simulink model "sampleModel7126_pp_1_1"  (R2018a)
settings: Solver=VariableStepAuto  StartTime=0.0  StopTime=10.0  RelTol=1e-3
undefined symbols (not defined in the file): DiscIntNeverNeededParam
libraries: simulink x367
(part 2 of 12)

== system sampleModel7126_pp_1_1/cfblk15 ==
  emi_1747 : Inport
  Action Port : ActionPort  ActionType=then
  cfblk15 : simulink/Continuous/PID Controller  Controller=PID  TimeDomain=Discrete-time  SampleTime=1  IntegratorMethod=Forward Euler  FilterMethod=Forward Euler  Form=Parallel  UseFilter=on  ControllerParametersSource=internal  P=1  I=1  D=0  N=100  InitialConditionSource=internal  InitialConditionForIntegrator=0  InitialConditionForFilter=0  ExternalReset=none  LimitOutput=off  UpperSaturationLimit=inf  LowerSaturationLimit=-inf  LinearizeAsGain=off  AntiWindupMode=none  Kb=1  TrackingMode=off  Kt=1  PParamMin=[]  PParamMax=[]  IParamMin=[]  IParamMax=[]  DParamMin=[]  DParamMax=[]  NParamMin=[]  NParamMax=[]  KbParamMin=[]  KbParamMax=[]  KtParamMin=[]  KtParamMax=[]  POutMin=[]  POutMax=[]  IOutMin=[]  IOutMax=[]  DOutMin=[]  DOutMax=[]  NOutMin=[]  NOutMax=[]  KbOutMin=[]  KbOutMax=[]  KtOutMin=[]  KtOutMax=[]  IntegratorOutMin=[]  IntegratorOutMax=[]  FilterOutMin=[]  FilterOutMax=[]  SumOutMin=[]  SumOutMax=[]  SumI1OutMin=[]  SumI1OutMax=[]  SumI2OutMin=[]  SumI2OutMax=[]  SumI3OutMin=[]  SumI3OutMax=[]  SumDOutMin=[]  SumDOutMax=[]  SaturationOutMin=[]  SaturationOutMax=[]  IntegratorContinuousStateAttributes=''  IntegratorStateMustResolveToSignalObject=off  IntegratorRTWStateStorageClass=Auto  FilterContinuousStateAttributes=''  FilterStateMustResolveToSignalObject=off  FilterRTWStateStorageClass=Auto  DifferentiatorICPrevScaledInput=0  DifferentiatorOutMin=[]  DifferentiatorOutMax=[]  FilterDiffOutCoefMin=[]  FilterDiffOutCoefMax=[]  SumDenOutMin=[]  SumDenOutMax=[]  SumNumOutMin=[]  SumNumOutMax=[]  ReciprocalOutMin=[]  ReciprocalOutMax=[]  DivideOutMin=[]  DivideOutMax=[]  TunerSelectOption=Transfer Function Based (PID Tuner App)
  emi_1748 : Outport
  wires:
  emi_1747/1 -> cfblk15/1
  cfblk15/1 -> emi_1748/1

== system sampleModel7126_pp_1_1/cfblk20 ==
  emi_1949 : Inport
  emi_1950 : Inport  Port=2
  Action Port : ActionPort  ActionType=then
  cfblk20 : Delay  DelayLengthSource=Input port  SampleTime=1
      settings: InputPortMap=u0,p1
  emi_1951 : Outport
  wires:
  emi_1949/1 -> cfblk20/1
  emi_1950/1 -> cfblk20/2
  cfblk20/1 -> emi_1951/1

== system sampleModel7126_pp_1_1/cfblk21 ==
  emi_194 : Inport
  emi_195 : Inport  Port=2
  Action Port : ActionPort  ActionType=then
  cfblk21 : simulink/Continuous/PID Controller (2DOF)  Controller=PID  TimeDomain=Discrete-time  SampleTime=1  IntegratorMethod=Forward Euler  FilterMethod=Forward Euler  Form=Parallel  UseFilter=on  ControllerParametersSource=internal  P=1  I=1  D=0  N=100  b=1  c=1  InitialConditionSource=internal  InitialConditionForIntegrator=0  InitialConditionForFilter=0  ExternalReset=none  LimitOutput=off  UpperSaturationLimit=inf  LowerSaturationLimit=-inf  LinearizeAsGain=off  AntiWindupMode=none  Kb=1  TrackingMode=off  Kt=1  PParamMin=[]  PParamMax=[]  IParamMin=[]  IParamMax=[]  DParamMin=[]  DParamMax=[]  NParamMin=[]  NParamMax=[]  bParamMin=[]  bParamMax=[]  cParamMin=[]  cParamMax=[]  KbParamMin=[]  KbParamMax=[]  KtParamMin=[]  KtParamMax=[]  POutMin=[]  POutMax=[]  IOutMin=[]  IOutMax=[]  DOutMin=[]  DOutMax=[]  NOutMin=[]  NOutMax=[]  bOutMin=[]  bOutMax=[]  cOutMin=[]  cOutMax=[]  KbOutMin=[]  KbOutMax=[]  KtOutMin=[]  KtOutMax=[]  IntegratorOutMin=[]  IntegratorOutMax=[]  FilterOutMin=[]  FilterOutMax=[]  SumOutMin=[]  SumOutMax=[]  Sum1OutMin=[]  Sum1OutMax=[]  Sum2OutMin=[]  Sum2OutMax=[]  Sum3OutMin=[]  Sum3OutMax=[]  SumI1OutMin=[]  SumI1OutMax=[]  SumI2OutMin=[]  SumI2OutMax=[]  SumI3OutMin=[]  SumI3OutMax=[]  SumDOutMin=[]  SumDOutMax=[]  SaturationOutMin=[]  SaturationOutMax=[]  IntegratorContinuousStateAttributes=''  IntegratorStateMustResolveToSignalObject=off  IntegratorRTWStateStorageClass=Auto  FilterContinuousStateAttributes=''  FilterStateMustResolveToSignalObject=off  FilterRTWStateStorageClass=Auto  DifferentiatorICPrevScaledInput=0  DifferentiatorOutMin=[]  DifferentiatorOutMax=[]  FilterDiffOutCoefMin=[]  FilterDiffOutCoefMax=[]  SumDenOutMin=[]  SumDenOutMax=[]  SumNumOutMin=[]  SumNumOutMax=[]  ReciprocalOutMin=[]  ReciprocalOutMax=[]  DivideOutMin=[]  DivideOutMax=[]  TunerSelectOption=Transfer Function Based (PID Tuner App)
  emi_196 : Outport
  wires:
  emi_194/1 -> cfblk21/1
  emi_195/1 -> cfblk21/2
  cfblk21/1 -> emi_196/1

== system sampleModel7126_pp_1_1/cfblk245 ==
  cfblk1 : Inport
  cfblk11 : Inport  Port=2
  cfblk12 : Inport  Port=3
  cfblk13 : Inport  Port=4
  cfblk14 : Inport  Port=5
  cfblk15 : Inport  Port=6
  Action Port : ActionPort  ActionType=then
  cfblk10 : If  SampleTime=1
  cfblk18 : Subsystem  TreatAsAtomicUnit=on
  cfblk19 : Subsystem  TreatAsAtomicUnit=on
  cfblk20 : Delay
  cfblk21 : DataTypeConversion  OutDataTypeStr=double
  cfblk3 : DiscreteIntegrator  SampleTime=-1  OutDataTypeStr=double  ICPrevOutput=DiscIntNeverNeededParam  ICPrevScaledInput=DiscIntNeverNeededParam
  cfblk4 : UnitDelay  SampleTime=-1
  cfblk5 : DiscreteZeroPole  Poles=[0 0.5]  Gain=1  SampleTime=-1
  cfblk6 : DiscreteFilter
  cfblk7 : simulink/Discrete/Transfer Fcn Real Zero  ZeroZ=0.75  ICPrevInput=0.0  DoSatur=off
      settings: SourceProductName=Simulink  SourceProductBaseCode=SL
  cfblk8 : Subsystem  TreatAsAtomicUnit=on
  cfblk9 : Delay
  cyemi_{68..70,79,90,92..98} (12 alike) : DataTypeConversion  OutDataTypeStr=double
  cyemi_91 : DataTypeConversion  OutDataTypeStr=fixdt('ufix32_En8')
  emi_671 : Subsystem  TreatAsAtomicUnit=on
  emi_673 : If  IfExpression=Inf <= u1  SampleTime=[1 0]
  emi_674 : DataTypeConversion  OutDataTypeStr=double
  cfblk2 : Outport
  cfblk16 : Outport  Port=2
  cfblk17 : Outport  Port=3
  wires:
  cfblk4/1 -> cfblk16/1, emi_674/1
  cfblk14/1 -> cfblk2/1
  cfblk18/3(cfblk11) -> cfblk17/1
  cfblk10/1 -> cfblk18/Action
  cfblk10/2 -> cfblk19/Action
  cyemi_68/1 -> cfblk10/1
  cfblk11/1 -> cyemi_68/1
  cyemi_69/1 -> cfblk18/1(cfblk1)
  cfblk15/1 -> cyemi_69/1
  cyemi_70/1 -> cfblk18/2(cfblk9)
  cfblk19/3(cfblk12) -> cyemi_70/1
  cyemi_79/1 -> cfblk19/1(cfblk1)
  cfblk3/1 -> cyemi_79/1
  cyemi_90/1 -> cfblk20/1
  cfblk18/2(cfblk10) -> cyemi_90/1
  cyemi_91/1 -> cfblk21/1
  cfblk1/1 -> cyemi_91/1
  cyemi_92/1 -> cfblk3/1
  cfblk20/1 -> cyemi_92/1
  cyemi_93/1 -> cfblk4/1
  cfblk7/1 -> cyemi_93/1
  cyemi_94/1 -> cfblk5/1
  cfblk21/1 -> cyemi_94/1
  cyemi_95/1 -> cfblk6/1
  cfblk19/1(cfblk2) -> cyemi_95/1
  cyemi_96/1 -> cfblk7/1
  cfblk18/1(cfblk2) -> cyemi_96/1
  cfblk19/2(cfblk11) -> cyemi_97/1
  cyemi_98/1 -> cfblk9/1
  cyemi_97/1 -> cfblk8/1(emi_669)
  cfblk8/1(emi_670) -> cyemi_98/1
  emi_673/1 -> cfblk8/Action
  emi_673/2 -> emi_671/Action
  emi_674/1 -> emi_673/1

== system sampleModel7126_pp_1_1/cfblk246 ==
  cfblk1 : Inport
  cfblk8 : Inport  Port=2
  Action Port : ActionPort  ActionType=else
  cfblk10 : Subsystem  TreatAsAtomicUnit=on
  cfblk11 : Delay
  cfblk3 : DiscreteFilter
  cfblk4 : Subsystem  TreatAsAtomicUnit=on
  cfblk5 : Subsystem  TreatAsAtomicUnit=on
  cfblk6 : simulink/Discrete/Transfer Fcn Lead or Lag  PoleZ=0.95  ZeroZ=0.75  ICPrevOutput=0.0  ICPrevInput=0.0  DoSatur=off
      settings: SourceProductName=Simulink  SourceProductBaseCode=SL
  cfblk7 : If  SampleTime=1
  cfblk9 : Subsystem  TreatAsAtomicUnit=on
  cyemi_{101..102,118..124} (9 alike) : DataTypeConversion  OutDataTypeStr=double
  emi_1864 : Subsystem  TreatAsAtomicUnit=on
  emi_1866 : If  IfExpression=0 <= u1  SampleTime=[1 0]
  emi_1867 : DataTypeConversion  OutDataTypeStr=double
  emi_515 : Subsystem  TreatAsAtomicUnit=on
  emi_517 : If  IfExpression=0 <= u1  SampleTime=[1 0]
  emi_518 : DataTypeConversion  OutDataTypeStr=double
  cfblk2 : Outport
  wires:
  cfblk6/1 -> cfblk2/1
  cfblk7/1 -> cfblk9/Action
  cfblk7/2 -> cfblk10/Action
  cyemi_101/1 -> cfblk10/1(cfblk1)
  cfblk11/1 -> cyemi_101/1
  cyemi_102/1 -> cfblk10/2(cfblk13)
  cfblk8/1 -> cyemi_102/1
  cyemi_118/1 -> cfblk11/1
  cyemi_119/1 -> cfblk3/1
  cfblk1/1 -> cyemi_119/1
  cfblk10/1(cfblk2) -> cyemi_120/1
  cfblk3/1 -> cyemi_121/1, emi_518/1
  cyemi_122/1 -> cfblk6/1
  cfblk10/3(cfblk15) -> cyemi_122/1
  cyemi_123/1 -> cfblk7/1
  cyemi_124/1 -> cfblk9/1(cfblk1)
  cfblk10/2(cfblk14) -> cyemi_124/1
  cyemi_120/1 -> cfblk4/1(emi_513)
  cfblk4/1(emi_514) -> cyemi_118/1, emi_1867/1
  emi_517/1 -> cfblk4/Action
  emi_517/2 -> emi_515/Action
  emi_518/1 -> emi_517/1
  cyemi_121/1 -> cfblk5/1(emi_1862)
  cfblk5/1(emi_1863) -> cyemi_123/1
  emi_1866/1 -> cfblk5/Action
  emi_1866/2 -> emi_1864/Action
  emi_1867/1 -> emi_1866/1

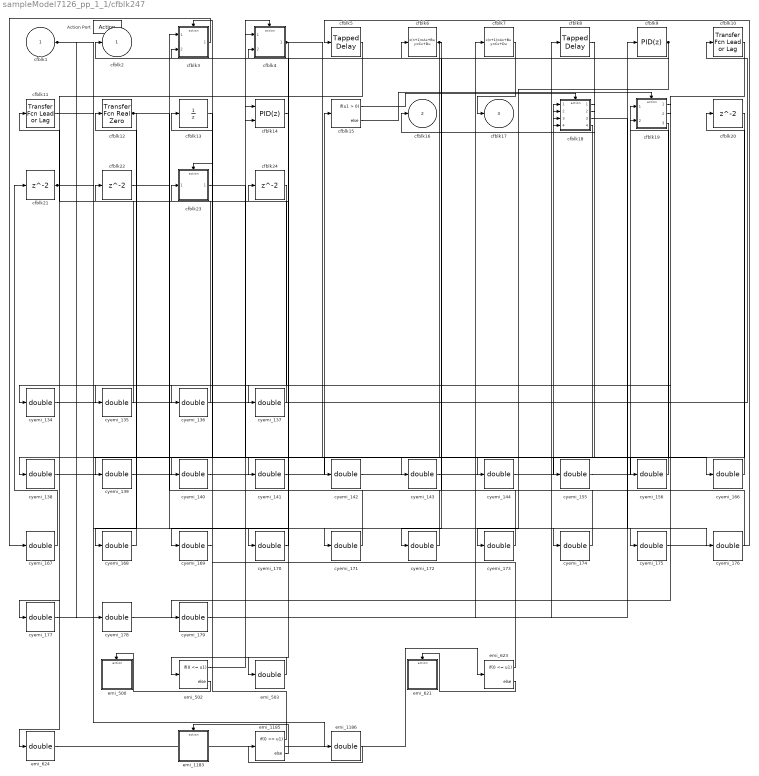
== system sampleModel7126_pp_1_1/cfblk247 ==
  cfblk1 : Inport
  Action Port : ActionPort  ActionType=then
  cfblk10 : simulink/Discrete/Transfer Fcn Lead or Lag  PoleZ=0.95  ZeroZ=0.75  ICPrevOutput=0.0  ICPrevInput=0.0  DoSatur=off
      settings: SourceProductName=Simulink  SourceProductBaseCode=SL
  cfblk11 : simulink/Discrete/Transfer Fcn Lead or Lag  PoleZ=0.95  ZeroZ=0.75  ICPrevOutput=0.0  ICPrevInput=0.0  DoSatur=off
      settings: SourceProductName=Simulink  SourceProductBaseCode=SL
  cfblk12 : simulink/Discrete/Transfer Fcn Real Zero  ZeroZ=0.75  ICPrevInput=0.0  DoSatur=off
      settings: SourceProductName=Simulink  SourceProductBaseCode=SL
  cfblk13 : UnitDelay  SampleTime=-1
  cfblk14 : simulink/Continuous/PID Controller (2DOF)  Controller=PID  TimeDomain=Discrete-time  SampleTime=-1  IntegratorMethod=Forward Euler  FilterMethod=Forward Euler  Form=Parallel  UseFilter=on  ControllerParametersSource=internal  P=1  I=1  D=0  N=100  b=1  c=1  InitialConditionSource=internal  InitialConditionForIntegrator=0  InitialConditionForFilter=0  ExternalReset=none  LimitOutput=off  UpperSaturationLimit=inf  LowerSaturationLimit=-inf  LinearizeAsGain=off  AntiWindupMode=none  Kb=1  TrackingMode=off  Kt=1  PParamMin=[]  PParamMax=[]  IParamMin=[]  IParamMax=[]  DParamMin=[]  DParamMax=[]  NParamMin=[]  NParamMax=[]  bParamMin=[]  bParamMax=[]  cParamMin=[]  cParamMax=[]  KbParamMin=[]  KbParamMax=[]  KtParamMin=[]  KtParamMax=[]  POutMin=[]  POutMax=[]  IOutMin=[]  IOutMax=[]  DOutMin=[]  DOutMax=[]  NOutMin=[]  NOutMax=[]  bOutMin=[]  bOutMax=[]  cOutMin=[]  cOutMax=[]  KbOutMin=[]  KbOutMax=[]  KtOutMin=[]  KtOutMax=[]  IntegratorOutMin=[]  IntegratorOutMax=[]  FilterOutMin=[]  FilterOutMax=[]  SumOutMin=[]  SumOutMax=[]  Sum1OutMin=[]  Sum1OutMax=[]  Sum2OutMin=[]  Sum2OutMax=[]  Sum3OutMin=[]  Sum3OutMax=[]  SumI1OutMin=[]  SumI1OutMax=[]  SumI2OutMin=[]  SumI2OutMax=[]  SumI3OutMin=[]  SumI3OutMax=[]  SumDOutMin=[]  SumDOutMax=[]  SaturationOutMin=[]  SaturationOutMax=[]  IntegratorContinuousStateAttributes=''  IntegratorStateMustResolveToSignalObject=off  IntegratorRTWStateStorageClass=Auto  FilterContinuousStateAttributes=''  FilterStateMustResolveToSignalObject=off  FilterRTWStateStorageClass=Auto  DifferentiatorICPrevScaledInput=0  DifferentiatorOutMin=[]  DifferentiatorOutMax=[]  FilterDiffOutCoefMin=[]  FilterDiffOutCoefMax=[]  SumDenOutMin=[]  SumDenOutMax=[]  SumNumOutMin=[]  SumNumOutMax=[]  ReciprocalOutMin=[]  ReciprocalOutMax=[]  DivideOutMin=[]  DivideOutMax=[]  TunerSelectOption=Transfer Function Based (PID Tuner App)
  cfblk15 : If  SampleTime=1
  cfblk18 : Subsystem  TreatAsAtomicUnit=on
  cfblk19 : Subsystem  TreatAsAtomicUnit=on
  cfblk{20..22,24} (4 alike) : Delay
  cfblk23 : Subsystem  TreatAsAtomicUnit=on
  cfblk3 : Subsystem  TreatAsAtomicUnit=on
  cfblk4 : Subsystem  TreatAsAtomicUnit=on
  cfblk5 : simulink/Discrete/Tapped Delay  vinit=0.0  samptime=-1  NumDelays=1  DelayOrder=Oldest  includeCurrent=off
  cfblk6 : DiscreteStateSpace  SampleTime=-1
  cfblk7 : DiscreteStateSpace  SampleTime=-1
  cfblk8 : simulink/Discrete/Tapped Delay  vinit=0.0  samptime=-1  NumDelays=1  DelayOrder=Oldest  includeCurrent=off
  cfblk9 : simulink/Continuous/PID Controller  Controller=PID  TimeDomain=Discrete-time  SampleTime=-1  IntegratorMethod=Forward Euler  FilterMethod=Forward Euler  Form=Parallel  UseFilter=on  ControllerParametersSource=internal  P=1  I=1  D=0  N=100  InitialConditionSource=internal  InitialConditionForIntegrator=0  InitialConditionForFilter=0  ExternalReset=none  LimitOutput=off  UpperSaturationLimit=inf  LowerSaturationLimit=-inf  LinearizeAsGain=off  AntiWindupMode=none  Kb=1  TrackingMode=off  Kt=1  PParamMin=[]  PParamMax=[]  IParamMin=[]  IParamMax=[]  DParamMin=[]  DParamMax=[]  NParamMin=[]  NParamMax=[]  KbParamMin=[]  KbParamMax=[]  KtParamMin=[]  KtParamMax=[]  POutMin=[]  POutMax=[]  IOutMin=[]  IOutMax=[]  DOutMin=[]  DOutMax=[]  NOutMin=[]  NOutMax=[]  KbOutMin=[]  KbOutMax=[]  KtOutMin=[]  KtOutMax=[]  IntegratorOutMin=[]  IntegratorOutMax=[]  FilterOutMin=[]  FilterOutMax=[]  SumOutMin=[]  SumOutMax=[]  SumI1OutMin=[]  SumI1OutMax=[]  SumI2OutMin=[]  SumI2OutMax=[]  SumI3OutMin=[]  SumI3OutMax=[]  SumDOutMin=[]  SumDOutMax=[]  SaturationOutMin=[]  SaturationOutMax=[]  IntegratorContinuousStateAttributes=''  IntegratorStateMustResolveToSignalObject=off  IntegratorRTWStateStorageClass=Auto  FilterContinuousStateAttributes=''  FilterStateMustResolveToSignalObject=off  FilterRTWStateStorageClass=Auto  DifferentiatorICPrevScaledInput=0  DifferentiatorOutMin=[]  DifferentiatorOutMax=[]  FilterDiffOutCoefMin=[]  FilterDiffOutCoefMax=[]  SumDenOutMin=[]  SumDenOutMax=[]  SumNumOutMin=[]  SumNumOutMax=[]  ReciprocalOutMin=[]  ReciprocalOutMax=[]  DivideOutMin=[]  DivideOutMax=[]  TunerSelectOption=Transfer Function Based (PID Tuner App)
  cyemi_{134..144,155..156,166..179} (27 alike) : DataTypeConversion  OutDataTypeStr=double
  emi_1183 : Subsystem  TreatAsAtomicUnit=on
  emi_1185 : If  IfExpression=0 <= u1  SampleTime=[1 0]
  emi_1186 : DataTypeConversion  OutDataTypeStr=double
  emi_500 : Subsystem  TreatAsAtomicUnit=on
  emi_502 : If  IfExpression=0 <= u1  SampleTime=[0 1]
  emi_503 : DataTypeConversion  OutDataTypeStr=double
  emi_621 : Subsystem  TreatAsAtomicUnit=on
  emi_623 : If  IfExpression=0 <= u1  SampleTime=[1 0]
  emi_624 : DataTypeConversion  OutDataTypeStr=double
  cfblk2 : Outport
  cfblk16 : Outport  Port=2
  cfblk17 : Outport  Port=3
  wires:
  cfblk1/1 -> cyemi_174/1, cyemi_178/1
  cfblk12/1 -> cyemi_168/1, cyemi_171/1
  cfblk18/2(cfblk14) -> cfblk16/1
  cfblk7/1 -> cfblk17/1
  cfblk9/1 -> cfblk2/1, cyemi_173/1
  cfblk15/1 -> cfblk18/Action
  cfblk15/2 -> cfblk19/Action
  cyemi_134/1 -> cfblk10/1
  cfblk19/1(cfblk2) -> cyemi_134/1
  cyemi_135/1 -> cfblk11/1
  cfblk18/1(cfblk2) -> cyemi_135/1
  cyemi_136/1 -> cfblk12/1
  cfblk13/1 -> cyemi_136/1
  cyemi_137/1 -> cfblk13/1
  cfblk14/1 -> cyemi_137/1
  cyemi_138/1 -> cfblk14/1
  cfblk5/1 -> cyemi_138/1
  cyemi_139/1 -> cfblk14/2
  cyemi_140/1 -> cfblk15/1
  cfblk24/1 -> cyemi_140/1
  cyemi_141/1 -> cfblk18/1(cfblk1)
  cfblk20/1 -> cyemi_141/1
  cyemi_142/1 -> cfblk18/2(cfblk11)
  cfblk19/2(cfblk12) -> cyemi_142/1
  cyemi_143/1 -> cfblk18/3(cfblk12)
  cfblk22/1 -> cyemi_143/1
  cyemi_144/1 -> cfblk18/4(cfblk13)
  cyemi_155/1 -> cfblk19/1(cfblk1)
  cfblk8/1 -> cyemi_155/1
  cyemi_156/1 -> cfblk19/2(cfblk11)
  cfblk21/1 -> cyemi_156/1, emi_624/1, emi_1186/1
  cyemi_166/1 -> cfblk20/1
  cyemi_167/1 -> cfblk21/1
  cyemi_168/1 -> cfblk22/1
  cyemi_170/1 -> cfblk24/1
  cfblk19/3(cfblk13) -> cyemi_170/1
  cfblk6/1 -> cyemi_172/1, emi_503/1
  cyemi_175/1 -> cfblk5/1
  cfblk11/1 -> cyemi_175/1
  cyemi_176/1 -> cfblk6/1
  cfblk18/3(cfblk15) -> cyemi_176/1
  cyemi_177/1 -> cfblk7/1
  cfblk18/4(cfblk16) -> cyemi_177/1
  cyemi_178/1 -> cfblk8/1
  cyemi_179/1 -> cfblk9/1
  cfblk10/1 -> cyemi_179/1
  cyemi_173/1 -> cfblk4/1(emi_497)
  cyemi_174/1 -> cfblk4/2(emi_498)
  cfblk4/1(emi_499) -> cyemi_169/1, cyemi_166/1, cyemi_139/1
  emi_502/1 -> cfblk4/Action
  emi_502/2 -> emi_500/Action
  emi_503/1 -> emi_502/1
  cyemi_169/1 -> cfblk23/1(emi_619)
  cfblk23/1(emi_620) -> cyemi_144/1
  emi_623/1 -> cfblk23/Action
  emi_623/2 -> emi_621/Action
  emi_624/1 -> emi_623/1
  cyemi_171/1 -> cfblk3/1(emi_1180)
  cyemi_172/1 -> cfblk3/2(emi_1181)
  cfblk3/1(emi_1182) -> cyemi_167/1
  emi_1185/1 -> cfblk3/Action
  emi_1185/2 -> emi_1183/Action
  emi_1186/1 -> emi_1185/1

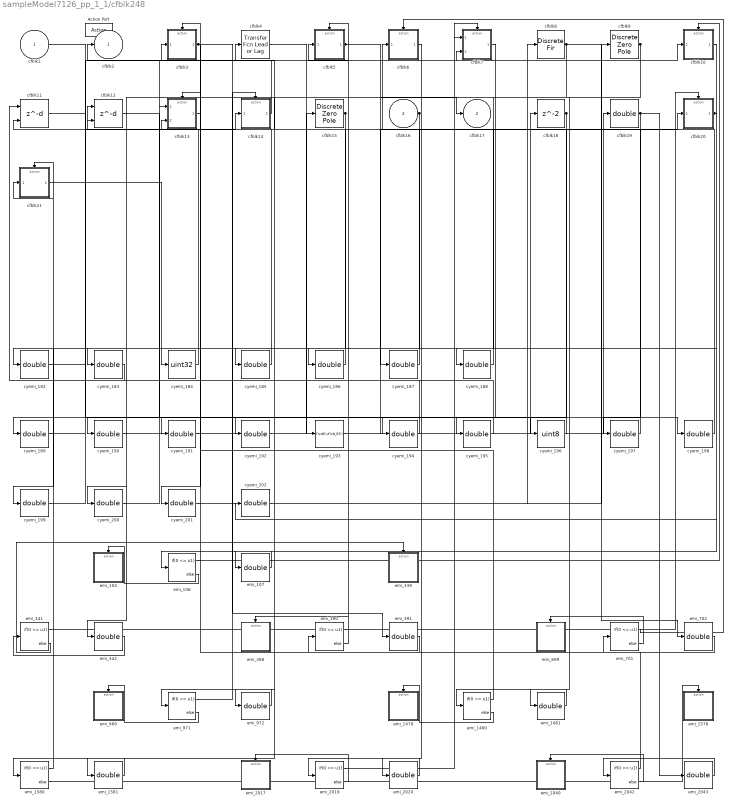
== system sampleModel7126_pp_1_1/cfblk248 ==
  cfblk1 : Inport
  cfblk16 : Inport  Port=2
  Action Port : ActionPort  ActionType=else
  cfblk10 : Subsystem  TreatAsAtomicUnit=on
  cfblk11 : Delay  DelayLengthSource=Input port
      settings: InputPortMap=u0,p1
  cfblk12 : Delay  DelayLengthSource=Input port
      settings: InputPortMap=u0,p1
  cfblk13 : Subsystem  TreatAsAtomicUnit=on
  cfblk14 : Subsystem  TreatAsAtomicUnit=on
  cfblk15 : DiscreteZeroPole  Poles=[0 0.5]  Gain=1  SampleTime=-1
  cfblk18 : Delay
  cfblk19 : DataTypeConversion  OutDataTypeStr=double
  cfblk20 : Subsystem  TreatAsAtomicUnit=on
  cfblk21 : Subsystem  TreatAsAtomicUnit=on
  cfblk3 : Subsystem  TreatAsAtomicUnit=on
  cfblk4 : simulink/Discrete/Transfer Fcn Lead or Lag  PoleZ=0.95  ZeroZ=0.75  ICPrevOutput=0.0  ICPrevInput=0.0  DoSatur=off
      settings: SourceProductName=Simulink  SourceProductBaseCode=SL
  cfblk5 : Subsystem  TreatAsAtomicUnit=on
  cfblk6 : Subsystem  TreatAsAtomicUnit=on
  cfblk7 : Subsystem  TreatAsAtomicUnit=on
  cfblk8 : DiscreteFir
  cfblk9 : DiscreteZeroPole  Poles=[0 0.5]  Gain=1  SampleTime=-1
  cyemi_{182..183,185..192,194..195,197..202} (18 alike) : DataTypeConversion  OutDataTypeStr=double
  cyemi_184 : DataTypeConversion  OutDataTypeStr=uint32
  cyemi_193 : DataTypeConversion  OutDataTypeStr=fixdt('ufix8_E3')
  cyemi_196 : DataTypeConversion  OutDataTypeStr=uint8
  emi_104 : Subsystem  TreatAsAtomicUnit=on
  emi_106 : If  IfExpression=0 <= u1
  emi_{107,342,391,702,972,1481,1581,2020,2043} (9 alike) : DataTypeConversion  OutDataTypeStr=double
  emi_1478 : Subsystem  TreatAsAtomicUnit=on
  emi_{341,971,1480,1580,2042} (5 alike) : If  IfExpression=0 <= u1  SampleTime=[1 0]
  emi_1578 : Subsystem  TreatAsAtomicUnit=on
  emi_2017 : Subsystem  TreatAsAtomicUnit=on
  emi_2019 : If  IfExpression=0 <= u1  SampleTime=[0 1]
  emi_2040 : Subsystem  TreatAsAtomicUnit=on
  emi_339 : Subsystem  TreatAsAtomicUnit=on
  emi_388 : Subsystem  TreatAsAtomicUnit=on
  emi_390 : If  IfExpression=0 <= u1  SampleTime=[0.1 0]
  emi_699 : Subsystem  TreatAsAtomicUnit=on
  emi_701 : If  IfExpression=0 <= u1  SampleTime=[0 1]
  emi_969 : Subsystem  TreatAsAtomicUnit=on
  cfblk2 : Outport
  cfblk17 : Outport  Port=2
  wires:
  cfblk9/1 -> cyemi_190/1, cyemi_200/1, emi_1481/1, emi_1581/1
  cfblk16/1 -> cyemi_182/1, cyemi_186/1
  cfblk8/1 -> cyemi_185/1, cyemi_188/1, emi_702/1
  cyemi_183/1 -> cfblk11/1
  cyemi_184/1 -> cfblk11/2
  cyemi_185/1 -> cfblk12/1
  cyemi_186/1 -> cfblk12/2
  cyemi_190/1 -> cfblk15/1
  cyemi_191/1 -> cfblk18/1
  cyemi_192/1 -> cfblk19/1
  cfblk11/1 -> cyemi_192/1
  cfblk4/1 -> cyemi_193/1
  cfblk18/1 -> cyemi_195/1, emi_342/1, emi_2020/1
  cyemi_196/1 -> cfblk4/1
  cfblk1/1 -> cyemi_196/1
  cfblk19/1 -> cyemi_197/1, emi_2043/1
  cfblk12/1 -> cyemi_198/1
  cfblk15/1 -> cyemi_199/1, emi_972/1
  cyemi_201/1 -> cfblk8/1
  cyemi_202/1 -> cfblk9/1
  cyemi_182/1 -> cfblk10/1(emi_102)
  cfblk10/1(emi_103) -> cyemi_202/1
  emi_106/1 -> cfblk10/Action
  emi_106/2 -> emi_104/Action
  emi_107/1 -> emi_106/1
  cyemi_193/1 -> cfblk20/1(emi_337)
  cfblk20/1(emi_338) -> emi_107/1, cyemi_183/1
  emi_341/1 -> cfblk20/Action
  emi_341/2 -> emi_339/Action
  emi_342/1 -> emi_341/1
  cyemi_197/1 -> cfblk5/1(emi_386)
  cfblk5/1(emi_387) -> cyemi_187/1, cfblk17/1
  emi_390/1 -> cfblk5/Action
  emi_390/2 -> emi_388/Action
  emi_391/1 -> emi_390/1
  cyemi_198/1 -> cfblk6/1(emi_697)
  cfblk6/1(emi_698) -> cyemi_191/1
  emi_701/1 -> cfblk6/Action
  emi_701/2 -> emi_699/Action
  emi_702/1 -> emi_701/1
  cyemi_189/1 -> cfblk14/1(emi_967)
  cfblk14/1(emi_968) -> cfblk2/1
  emi_971/1 -> cfblk14/Action
  emi_971/2 -> emi_969/Action
  emi_972/1 -> emi_971/1
  cyemi_195/1 -> cfblk3/1(emi_1476)
  cfblk3/1(emi_1477) -> emi_391/1, cyemi_201/1
  emi_1480/1 -> cfblk3/Action
  emi_1480/2 -> emi_1478/Action
  emi_1481/1 -> emi_1480/1
  cyemi_194/1 -> cfblk21/1(emi_1576)
  cfblk21/1(emi_1577) -> cyemi_184/1
  emi_1580/1 -> cfblk21/Action
  emi_1580/2 -> emi_1578/Action
  emi_1581/1 -> emi_1580/1
  cyemi_199/1 -> cfblk7/1(emi_2014)
  cyemi_200/1 -> cfblk7/2(emi_2015)
  cfblk7/1(emi_2016) -> cyemi_194/1
  emi_2019/1 -> cfblk7/Action
  emi_2019/2 -> emi_2017/Action
  emi_2020/1 -> emi_2019/1
  cyemi_187/1 -> cfblk13/1(emi_2037)
  cyemi_188/1 -> cfblk13/2(emi_2038)
  cfblk13/1(emi_2039) -> cyemi_189/1
  emi_2042/1 -> cfblk13/Action
  emi_2042/2 -> emi_2040/Action
  emi_2043/1 -> emi_2042/1

== system sampleModel7126_pp_1_1/cfblk249 ==
  cfblk1 : Inport
  cfblk14 : Inport  Port=2
  cfblk15 : Inport  Port=3
  Action Port : ActionPort  ActionType=then
  cfblk10 : Subsystem  TreatAsAtomicUnit=on
  cfblk11 : simulink/Continuous/PID Controller (2DOF)  Controller=PID  TimeDomain=Discrete-time  SampleTime=-1  IntegratorMethod=Forward Euler  FilterMethod=Forward Euler  Form=Parallel  UseFilter=on  ControllerParametersSource=internal  P=1  I=1  D=0  N=100  b=1  c=1  InitialConditionSource=internal  InitialConditionForIntegrator=0  InitialConditionForFilter=0  ExternalReset=none  LimitOutput=off  UpperSaturationLimit=inf  LowerSaturationLimit=-inf  LinearizeAsGain=off  AntiWindupMode=none  Kb=1  TrackingMode=off  Kt=1  PParamMin=[]  PParamMax=[]  IParamMin=[]  IParamMax=[]  DParamMin=[]  DParamMax=[]  NParamMin=[]  NParamMax=[]  bParamMin=[]  bParamMax=[]  cParamMin=[]  cParamMax=[]  KbParamMin=[]  KbParamMax=[]  KtParamMin=[]  KtParamMax=[]  POutMin=[]  POutMax=[]  IOutMin=[]  IOutMax=[]  DOutMin=[]  DOutMax=[]  NOutMin=[]  NOutMax=[]  bOutMin=[]  bOutMax=[]  cOutMin=[]  cOutMax=[]  KbOutMin=[]  KbOutMax=[]  KtOutMin=[]  KtOutMax=[]  IntegratorOutMin=[]  IntegratorOutMax=[]  FilterOutMin=[]  FilterOutMax=[]  SumOutMin=[]  SumOutMax=[]  Sum1OutMin=[]  Sum1OutMax=[]  Sum2OutMin=[]  Sum2OutMax=[]  Sum3OutMin=[]  Sum3OutMax=[]  SumI1OutMin=[]  SumI1OutMax=[]  SumI2OutMin=[]  SumI2OutMax=[]  SumI3OutMin=[]  SumI3OutMax=[]  SumDOutMin=[]  SumDOutMax=[]  SaturationOutMin=[]  SaturationOutMax=[]  IntegratorContinuousStateAttributes=''  IntegratorStateMustResolveToSignalObject=off  IntegratorRTWStateStorageClass=Auto  FilterContinuousStateAttributes=''  FilterStateMustResolveToSignalObject=off  FilterRTWStateStorageClass=Auto  DifferentiatorICPrevScaledInput=0  DifferentiatorOutMin=[]  DifferentiatorOutMax=[]  FilterDiffOutCoefMin=[]  FilterDiffOutCoefMax=[]  SumDenOutMin=[]  SumDenOutMax=[]  SumNumOutMin=[]  SumNumOutMax=[]  ReciprocalOutMin=[]  ReciprocalOutMax=[]  DivideOutMin=[]  DivideOutMax=[]  TunerSelectOption=Transfer Function Based (PID Tuner App)
  cfblk12 : DiscreteZeroPole  Poles=[0 0.5]  Gain=1  SampleTime=-1
  cfblk13 : Delay  DelayLengthSource=Input port
      settings: InputPortMap=u0,p1
  cfblk17 : Delay
  cfblk3 : Subsystem  TreatAsAtomicUnit=on
  cfblk4 : simulink/Continuous/PID Controller  Controller=PID  TimeDomain=Discrete-time  SampleTime=-1  IntegratorMethod=Forward Euler  FilterMethod=Forward Euler  Form=Parallel  UseFilter=on  ControllerParametersSource=internal  P=1  I=1  D=0  N=100  InitialConditionSource=internal  InitialConditionForIntegrator=0  InitialConditionForFilter=0  ExternalReset=none  LimitOutput=off  UpperSaturationLimit=inf  LowerSaturationLimit=-inf  LinearizeAsGain=off  AntiWindupMode=none  Kb=1  TrackingMode=off  Kt=1  PParamMin=[]  PParamMax=[]  IParamMin=[]  IParamMax=[]  DParamMin=[]  DParamMax=[]  NParamMin=[]  NParamMax=[]  KbParamMin=[]  KbParamMax=[]  KtParamMin=[]  KtParamMax=[]  POutMin=[]  POutMax=[]  IOutMin=[]  IOutMax=[]  DOutMin=[]  DOutMax=[]  NOutMin=[]  NOutMax=[]  KbOutMin=[]  KbOutMax=[]  KtOutMin=[]  KtOutMax=[]  IntegratorOutMin=[]  IntegratorOutMax=[]  FilterOutMin=[]  FilterOutMax=[]  SumOutMin=[]  SumOutMax=[]  SumI1OutMin=[]  SumI1OutMax=[]  SumI2OutMin=[]  SumI2OutMax=[]  SumI3OutMin=[]  SumI3OutMax=[]  SumDOutMin=[]  SumDOutMax=[]  SaturationOutMin=[]  SaturationOutMax=[]  IntegratorContinuousStateAttributes=''  IntegratorStateMustResolveToSignalObject=off  IntegratorRTWStateStorageClass=Auto  FilterContinuousStateAttributes=''  FilterStateMustResolveToSignalObject=off  FilterRTWStateStorageClass=Auto  DifferentiatorICPrevScaledInput=0  DifferentiatorOutMin=[]  DifferentiatorOutMax=[]  FilterDiffOutCoefMin=[]  FilterDiffOutCoefMax=[]  SumDenOutMin=[]  SumDenOutMax=[]  SumNumOutMin=[]  SumNumOutMax=[]  ReciprocalOutMin=[]  ReciprocalOutMax=[]  DivideOutMin=[]  DivideOutMax=[]  TunerSelectOption=Transfer Function Based (PID Tuner App)
  cfblk5 : Subsystem  TreatAsAtomicUnit=on
  cfblk6 : simulink/Continuous/PID Controller  Controller=PID  TimeDomain=Discrete-time  SampleTime=-1  IntegratorMethod=Forward Euler  FilterMethod=Forward Euler  Form=Parallel  UseFilter=on  ControllerParametersSource=internal  P=1  I=1  D=0  N=100  InitialConditionSource=internal  InitialConditionForIntegrator=0  InitialConditionForFilter=0  ExternalReset=none  LimitOutput=off  UpperSaturationLimit=inf  LowerSaturationLimit=-inf  LinearizeAsGain=off  AntiWindupMode=none  Kb=1  TrackingMode=off  Kt=1  PParamMin=[]  PParamMax=[]  IParamMin=[]  IParamMax=[]  DParamMin=[]  DParamMax=[]  NParamMin=[]  NParamMax=[]  KbParamMin=[]  KbParamMax=[]  KtParamMin=[]  KtParamMax=[]  POutMin=[]  POutMax=[]  IOutMin=[]  IOutMax=[]  DOutMin=[]  DOutMax=[]  NOutMin=[]  NOutMax=[]  KbOutMin=[]  KbOutMax=[]  KtOutMin=[]  KtOutMax=[]  IntegratorOutMin=[]  IntegratorOutMax=[]  FilterOutMin=[]  FilterOutMax=[]  SumOutMin=[]  SumOutMax=[]  SumI1OutMin=[]  SumI1OutMax=[]  SumI2OutMin=[]  SumI2OutMax=[]  SumI3OutMin=[]  SumI3OutMax=[]  SumDOutMin=[]  SumDOutMax=[]  SaturationOutMin=[]  SaturationOutMax=[]  IntegratorContinuousStateAttributes=''  IntegratorStateMustResolveToSignalObject=off  IntegratorRTWStateStorageClass=Auto  FilterContinuousStateAttributes=''  FilterStateMustResolveToSignalObject=off  FilterRTWStateStorageClass=Auto  DifferentiatorICPrevScaledInput=0  DifferentiatorOutMin=[]  DifferentiatorOutMax=[]  FilterDiffOutCoefMin=[]  FilterDiffOutCoefMax=[]  SumDenOutMin=[]  SumDenOutMax=[]  SumNumOutMin=[]  SumNumOutMax=[]  ReciprocalOutMin=[]  ReciprocalOutMax=[]  DivideOutMin=[]  DivideOutMax=[]  TunerSelectOption=Transfer Function Based (PID Tuner App)
  cfblk7 : Delay  DelayLengthSource=Input port
      settings: InputPortMap=u0,p1
  cfblk8 : DiscreteFir
  cfblk9 : Subsystem  TreatAsAtomicUnit=on
  cyemi_{206..221} (16 alike) : DataTypeConversion  OutDataTypeStr=double
  emi_1787 : Subsystem  TreatAsAtomicUnit=on
  emi_1789 : If  IfExpression=Inf <= u1
  emi_{547,582,1790,2121} (4 alike) : DataTypeConversion  OutDataTypeStr=double
  emi_2118 : Subsystem  TreatAsAtomicUnit=on
  emi_2120 : If  IfExpression=Inf <= u1  SampleTime=[1 0]
  emi_544 : Subsystem  TreatAsAtomicUnit=on
  emi_546 : If  IfExpression=Inf <= u1  SampleTime=[1 0]
  emi_579 : Subsystem  TreatAsAtomicUnit=on
  emi_581 : If  IfExpression=Inf <= u1  SampleTime=[1 0]
  cfblk2 : Outport
  cfblk16 : Outport  Port=2
  wires:
  cfblk14/1 -> cyemi_216/1, cyemi_219/1
  cfblk11/1 -> cfblk2/1
  cfblk12/1 -> cyemi_212/1, cyemi_214/1, cyemi_220/1, emi_547/1
  cfblk6/1 -> cfblk16/1
  cfblk7/1 -> cyemi_207/1
  cyemi_208/1 -> cfblk11/1
  cyemi_209/1 -> cfblk11/2
  cyemi_210/1 -> cfblk12/1
  cyemi_211/1 -> cfblk13/1
  cfblk15/1 -> cyemi_211/1
  cyemi_212/1 -> cfblk13/2
  cyemi_213/1 -> cfblk17/1
  cfblk13/1 -> cyemi_213/1
  cyemi_215/1 -> cfblk4/1
  cfblk17/1 -> cyemi_215/1
  cyemi_217/1 -> cfblk6/1
  cfblk1/1 -> cyemi_217/1
  cyemi_218/1 -> cfblk7/1
  cfblk8/1 -> cyemi_218/1, emi_1790/1
  cyemi_219/1 -> cfblk7/2
  cyemi_220/1 -> cfblk8/1
  cfblk4/1 -> cyemi_221/1
  cyemi_216/1 -> cfblk5/1(emi_542)
  cfblk5/1(emi_543) -> cyemi_206/1, emi_582/1
  emi_546/1 -> cfblk5/Action
  emi_546/2 -> emi_544/Action
  emi_547/1 -> emi_546/1
  cyemi_221/1 -> cfblk9/1(emi_577)
  cfblk9/1(emi_578) -> cyemi_210/1, emi_2121/1
  emi_581/1 -> cfblk9/Action
  emi_581/2 -> emi_579/Action
  emi_582/1 -> emi_581/1
  cyemi_206/1 -> cfblk10/1(emi_1784)
  cyemi_207/1 -> cfblk10/2(emi_1785)
  cfblk10/1(emi_1786) -> cyemi_209/1
  emi_1789/1 -> cfblk10/Action
  emi_1789/2 -> emi_1787/Action
  emi_1790/1 -> emi_1789/1
  cyemi_214/1 -> cfblk3/1(emi_2116)
  cfblk3/1(emi_2117) -> cyemi_208/1
  emi_2120/1 -> cfblk3/Action
  emi_2120/2 -> emi_2118/Action
  emi_2121/1 -> emi_2120/1

== system sampleModel7126_pp_1_1/cfblk25 ==
  emi_662 : Inport
  Action Port : ActionPort  ActionType=then
  cfblk25 : simulink/Discrete/Transfer Fcn Real Zero  ZeroZ=0.75  ICPrevInput=0.0  DoSatur=off
      settings: SourceProductName=Simulink  SourceProductBaseCode=SL
  emi_663 : Outport
  wires:
  emi_662/1 -> cfblk25/1
  cfblk25/1 -> emi_663/1

== system sampleModel7126_pp_1_1/cfblk250 ==
  cfblk1 : Inport
  cfblk8 : Inport  Port=2
  Action Port : ActionPort  ActionType=else
  cfblk10 : Delay
  cfblk11 : Delay
  cfblk3 : simulink/Discrete/Transfer Fcn Real Zero  ZeroZ=0.75  ICPrevInput=0.0  DoSatur=off
      settings: SourceProductName=Simulink  SourceProductBaseCode=SL
  cfblk4 : Subsystem  TreatAsAtomicUnit=on
  cfblk5 : DiscreteZeroPole  Poles=[0 0.5]  Gain=1  SampleTime=-1
  cfblk6 : Subsystem  TreatAsAtomicUnit=on
  cfblk7 : Delay  DelayLengthSource=Input port
      settings: InputPortMap=u0,p1
  cyemi_{225..232} (8 alike) : DataTypeConversion  OutDataTypeStr=double
  emi_1315 : Subsystem  TreatAsAtomicUnit=on
  emi_1317 : If  IfExpression=0 <= u1  SampleTime=[1 0]
  emi_1318 : DataTypeConversion  OutDataTypeStr=double
  emi_1843 : Subsystem  TreatAsAtomicUnit=on
  emi_1845 : If  IfExpression=0 <= u1  SampleTime=[1 0]
  emi_1846 : DataTypeConversion  OutDataTypeStr=double
  cfblk2 : Outport
  cfblk9 : Outport  Port=2
  wires:
  cfblk1/1 -> cfblk2/1
  cfblk7/1 -> cyemi_225/1, cyemi_229/1, emi_1846/1
  cyemi_225/1 -> cfblk10/1
  cyemi_226/1 -> cfblk11/1
  cfblk5/1 -> cyemi_226/1, emi_1318/1
  cyemi_227/1 -> cfblk3/1
  cfblk10/1 -> cyemi_227/1
  cfblk3/1 -> cyemi_228/1
  cyemi_229/1 -> cfblk5/1
  cfblk8/1 -> cyemi_230/1
  cyemi_231/1 -> cfblk7/1
  cyemi_232/1 -> cfblk7/2
  cfblk11/1 -> cyemi_232/1
  cyemi_230/1 -> cfblk6/1(emi_1313)
  cfblk6/1(emi_1314) -> cfblk9/1
  emi_1317/1 -> cfblk6/Action
  emi_1317/2 -> emi_1315/Action
  emi_1318/1 -> emi_1317/1
  cyemi_228/1 -> cfblk4/1(emi_1841)
  cfblk4/1(emi_1842) -> cyemi_231/1
  emi_1845/1 -> cfblk4/Action
  emi_1845/2 -> emi_1843/Action
  emi_1846/1 -> emi_1845/1

== system sampleModel7126_pp_1_1/cfblk251 ==
  cfblk1 : Inport
  Action Port : ActionPort  ActionType=then
  cfblk10 : Delay
  cfblk12 : Delay
  cfblk3 : DiscreteStateSpace  SampleTime=-1
  cfblk4 : simulink/Discrete/Transfer Fcn Real Zero  ZeroZ=0.75  ICPrevInput=0.0  DoSatur=off
      settings: SourceProductName=Simulink  SourceProductBaseCode=SL
  cfblk5 : Subsystem  TreatAsAtomicUnit=on
  cfblk6 : Subsystem  TreatAsAtomicUnit=on
  cfblk7 : simulink/Discrete/Difference  ICPrevInput=0.0  OutMin=[]  OutMax=[]  OutDataTypeStr=double  OutputDataTypeScalingMode=double  OutDataType=fixdt(1, 16)  OutScaling=2^-10  DoSatur=off
  cfblk8 : simulink/Discrete/Transfer Fcn Lead or Lag  PoleZ=0.95  ZeroZ=0.75  ICPrevOutput=0.0  ICPrevInput=0.0  DoSatur=off
      settings: SourceProductName=Simulink  SourceProductBaseCode=SL
  cfblk9 : DiscreteIntegrator  SampleTime=-1  OutDataTypeStr=double  ICPrevOutput=DiscIntNeverNeededParam  ICPrevScaledInput=DiscIntNeverNeededParam
  cyemi_{234..242} (9 alike) : DataTypeConversion  OutDataTypeStr=double
  emi_1400 : Subsystem  TreatAsAtomicUnit=on
  emi_1402 : If  IfExpression=0 <= u1  SampleTime=[1 0]
  emi_1403 : DataTypeConversion  OutDataTypeStr=double
  emi_1492 : Subsystem  TreatAsAtomicUnit=on
  emi_1494 : If  IfExpression=0 <= u1  SampleTime=[1 0]
  emi_1495 : DataTypeConversion  OutDataTypeStr=double
  cfblk2 : Outport
  cfblk11 : Outport  Port=2
  wires:
  cfblk7/1 -> cyemi_237/1, cyemi_242/1
  cfblk8/1 -> cfblk11/1
  cfblk10/1 -> cfblk2/1, emi_1495/1
  cyemi_234/1 -> cfblk10/1
  cyemi_235/1 -> cfblk12/1
  cfblk9/1 -> cyemi_235/1, emi_1403/1
  cyemi_236/1 -> cfblk3/1
  cyemi_237/1 -> cfblk4/1
  cfblk4/1 -> cyemi_238/1
  cfblk1/1 -> cyemi_239/1
  cyemi_240/1 -> cfblk7/1
  cfblk12/1 -> cyemi_240/1
  cyemi_241/1 -> cfblk8/1
  cfblk3/1 -> cyemi_241/1
  cyemi_242/1 -> cfblk9/1
  cyemi_239/1 -> cfblk6/1(emi_1398)
  cfblk6/1(emi_1399) -> cyemi_234/1
  emi_1402/1 -> cfblk6/Action
  emi_1402/2 -> emi_1400/Action
  emi_1403/1 -> emi_1402/1
  cyemi_238/1 -> cfblk5/1(emi_1490)
  cfblk5/1(emi_1491) -> cyemi_236/1
  emi_1494/1 -> cfblk5/Action
  emi_1494/2 -> emi_1492/Action
  emi_1495/1 -> emi_1494/1

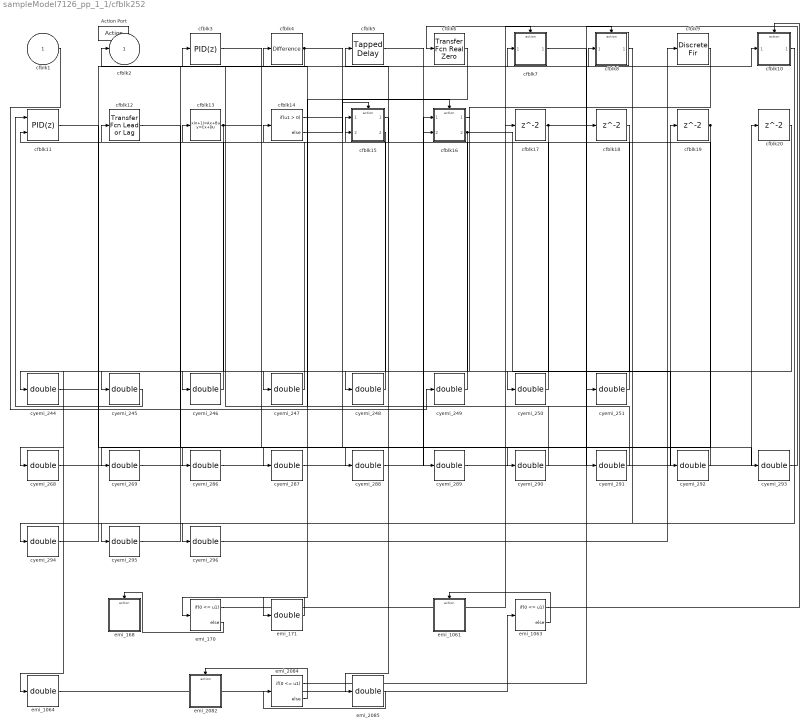
== system sampleModel7126_pp_1_1/cfblk252 ==
  cfblk1 : Inport
  Action Port : ActionPort  ActionType=else
  cfblk10 : Subsystem  TreatAsAtomicUnit=on
  cfblk11 : simulink/Continuous/PID Controller (2DOF)  Controller=PID  TimeDomain=Discrete-time  SampleTime=-1  IntegratorMethod=Forward Euler  FilterMethod=Forward Euler  Form=Parallel  UseFilter=on  ControllerParametersSource=internal  P=1  I=1  D=0  N=100  b=1  c=1  InitialConditionSource=internal  InitialConditionForIntegrator=0  InitialConditionForFilter=0  ExternalReset=none  LimitOutput=off  UpperSaturationLimit=inf  LowerSaturationLimit=-inf  LinearizeAsGain=off  AntiWindupMode=none  Kb=1  TrackingMode=off  Kt=1  PParamMin=[]  PParamMax=[]  IParamMin=[]  IParamMax=[]  DParamMin=[]  DParamMax=[]  NParamMin=[]  NParamMax=[]  bParamMin=[]  bParamMax=[]  cParamMin=[]  cParamMax=[]  KbParamMin=[]  KbParamMax=[]  KtParamMin=[]  KtParamMax=[]  POutMin=[]  POutMax=[]  IOutMin=[]  IOutMax=[]  DOutMin=[]  DOutMax=[]  NOutMin=[]  NOutMax=[]  bOutMin=[]  bOutMax=[]  cOutMin=[]  cOutMax=[]  KbOutMin=[]  KbOutMax=[]  KtOutMin=[]  KtOutMax=[]  IntegratorOutMin=[]  IntegratorOutMax=[]  FilterOutMin=[]  FilterOutMax=[]  SumOutMin=[]  SumOutMax=[]  Sum1OutMin=[]  Sum1OutMax=[]  Sum2OutMin=[]  Sum2OutMax=[]  Sum3OutMin=[]  Sum3OutMax=[]  SumI1OutMin=[]  SumI1OutMax=[]  SumI2OutMin=[]  SumI2OutMax=[]  SumI3OutMin=[]  SumI3OutMax=[]  SumDOutMin=[]  SumDOutMax=[]  SaturationOutMin=[]  SaturationOutMax=[]  IntegratorContinuousStateAttributes=''  IntegratorStateMustResolveToSignalObject=off  IntegratorRTWStateStorageClass=Auto  FilterContinuousStateAttributes=''  FilterStateMustResolveToSignalObject=off  FilterRTWStateStorageClass=Auto  DifferentiatorICPrevScaledInput=0  DifferentiatorOutMin=[]  DifferentiatorOutMax=[]  FilterDiffOutCoefMin=[]  FilterDiffOutCoefMax=[]  SumDenOutMin=[]  SumDenOutMax=[]  SumNumOutMin=[]  SumNumOutMax=[]  ReciprocalOutMin=[]  ReciprocalOutMax=[]  DivideOutMin=[]  DivideOutMax=[]  TunerSelectOption=Transfer Function Based (PID Tuner App)
  cfblk12 : simulink/Discrete/Transfer Fcn Lead or Lag  PoleZ=0.95  ZeroZ=0.75  ICPrevOutput=0.0  ICPrevInput=0.0  DoSatur=off
      settings: SourceProductName=Simulink  SourceProductBaseCode=SL
  cfblk13 : DiscreteStateSpace  SampleTime=-1
  cfblk14 : If  SampleTime=1
  cfblk15 : Subsystem  TreatAsAtomicUnit=on
  cfblk16 : Subsystem  TreatAsAtomicUnit=on
  cfblk{17..20} (4 alike) : Delay
  cfblk3 : simulink/Continuous/PID Controller  Controller=PID  TimeDomain=Discrete-time  SampleTime=-1  IntegratorMethod=Forward Euler  FilterMethod=Forward Euler  Form=Parallel  UseFilter=on  ControllerParametersSource=internal  P=1  I=1  D=0  N=100  InitialConditionSource=internal  InitialConditionForIntegrator=0  InitialConditionForFilter=0  ExternalReset=none  LimitOutput=off  UpperSaturationLimit=inf  LowerSaturationLimit=-inf  LinearizeAsGain=off  AntiWindupMode=none  Kb=1  TrackingMode=off  Kt=1  PParamMin=[]  PParamMax=[]  IParamMin=[]  IParamMax=[]  DParamMin=[]  DParamMax=[]  NParamMin=[]  NParamMax=[]  KbParamMin=[]  KbParamMax=[]  KtParamMin=[]  KtParamMax=[]  POutMin=[]  POutMax=[]  IOutMin=[]  IOutMax=[]  DOutMin=[]  DOutMax=[]  NOutMin=[]  NOutMax=[]  KbOutMin=[]  KbOutMax=[]  KtOutMin=[]  KtOutMax=[]  IntegratorOutMin=[]  IntegratorOutMax=[]  FilterOutMin=[]  FilterOutMax=[]  SumOutMin=[]  SumOutMax=[]  SumI1OutMin=[]  SumI1OutMax=[]  SumI2OutMin=[]  SumI2OutMax=[]  SumI3OutMin=[]  SumI3OutMax=[]  SumDOutMin=[]  SumDOutMax=[]  SaturationOutMin=[]  SaturationOutMax=[]  IntegratorContinuousStateAttributes=''  IntegratorStateMustResolveToSignalObject=off  IntegratorRTWStateStorageClass=Auto  FilterContinuousStateAttributes=''  FilterStateMustResolveToSignalObject=off  FilterRTWStateStorageClass=Auto  DifferentiatorICPrevScaledInput=0  DifferentiatorOutMin=[]  DifferentiatorOutMax=[]  FilterDiffOutCoefMin=[]  FilterDiffOutCoefMax=[]  SumDenOutMin=[]  SumDenOutMax=[]  SumNumOutMin=[]  SumNumOutMax=[]  ReciprocalOutMin=[]  ReciprocalOutMax=[]  DivideOutMin=[]  DivideOutMax=[]  TunerSelectOption=Transfer Function Based (PID Tuner App)
  cfblk4 : simulink/Discrete/Difference  ICPrevInput=0.0  OutMin=[]  OutMax=[]  OutDataTypeStr=double  OutputDataTypeScalingMode=double  OutDataType=fixdt(1, 16)  OutScaling=2^-10  DoSatur=off
  cfblk5 : simulink/Discrete/Tapped Delay  vinit=0.0  samptime=-1  NumDelays=1  DelayOrder=Oldest  includeCurrent=off
  cfblk6 : simulink/Discrete/Transfer Fcn Real Zero  ZeroZ=0.75  ICPrevInput=0.0  DoSatur=off
      settings: SourceProductName=Simulink  SourceProductBaseCode=SL
  cfblk7 : Subsystem  TreatAsAtomicUnit=on
  cfblk8 : Subsystem  TreatAsAtomicUnit=on
  cfblk9 : DiscreteFir
  cyemi_{244..251,268..269,286..296} (21 alike) : DataTypeConversion  OutDataTypeStr=double
  emi_1061 : Subsystem  TreatAsAtomicUnit=on
  emi_1063 : If  IfExpression=0 <= u1
  emi_1064 : DataTypeConversion  OutDataTypeStr=double
  emi_168 : Subsystem  TreatAsAtomicUnit=on
  emi_170 : If  IfExpression=0 <= u1  SampleTime=[0 1]
  emi_171 : DataTypeConversion  OutDataTypeStr=double
  emi_2082 : Subsystem  TreatAsAtomicUnit=on
  emi_2084 : If  IfExpression=0 <= u1  SampleTime=[1 0]
  emi_2085 : DataTypeConversion  OutDataTypeStr=double
  cfblk2 : Outport
  wires:
  cfblk16/2(cfblk17) -> cyemi_248/1, cyemi_292/1
  cfblk4/1 -> cfblk2/1, cyemi_293/1
  cfblk14/1 -> cfblk15/Action
  cfblk14/2 -> cfblk16/Action
  cfblk15/2(cfblk16) -> cyemi_244/1
  cyemi_245/1 -> cfblk11/1
  cfblk16/1(cfblk2) -> cyemi_245/1
  cyemi_246/1 -> cfblk11/2
  cfblk9/1 -> cyemi_246/1
  cyemi_247/1 -> cfblk12/1
  cfblk6/1 -> cyemi_247/1
  cyemi_248/1 -> cfblk13/1
  cyemi_249/1 -> cfblk14/1
  cfblk1/1 -> cyemi_249/1
  cyemi_250/1 -> cfblk15/1(cfblk1)
  cfblk20/1 -> cyemi_250/1
  cyemi_251/1 -> cfblk15/2(cfblk15)
  cfblk17/1 -> cyemi_251/1, emi_171/1
  cyemi_268/1 -> cfblk16/1(cfblk1)
  cfblk18/1 -> cyemi_268/1
  cyemi_269/1 -> cfblk16/2(cfblk16)
  cfblk19/1 -> cyemi_269/1, emi_2085/1
  cyemi_286/1 -> cfblk17/1
  cfblk11/1 -> cyemi_286/1
  cyemi_287/1 -> cfblk18/1
  cfblk12/1 -> cyemi_287/1
  cyemi_288/1 -> cfblk19/1
  cfblk3/1 -> cyemi_288/1
  cyemi_289/1 -> cfblk20/1
  cfblk5/1 -> cyemi_289/1
  cyemi_290/1 -> cfblk3/1
  cfblk13/1 -> cyemi_290/1, emi_1064/1
  cyemi_291/1 -> cfblk4/1
  cyemi_292/1 -> cfblk5/1
  cyemi_293/1 -> cfblk6/1
  cyemi_296/1 -> cfblk9/1
  cfblk15/1(cfblk2) -> cyemi_296/1
  cyemi_294/1 -> cfblk7/1(emi_166)
  cfblk7/1(emi_167) -> cyemi_291/1
  emi_170/1 -> cfblk7/Action
  emi_170/2 -> emi_168/Action
  emi_171/1 -> emi_170/1
  cyemi_244/1 -> cfblk10/1(emi_1059)
  cfblk10/1(emi_1060) -> cyemi_295/1
  emi_1063/1 -> cfblk10/Action
  emi_1063/2 -> emi_1061/Action
  emi_1064/1 -> emi_1063/1
  cyemi_295/1 -> cfblk8/1(emi_2080)
  cfblk8/1(emi_2081) -> cyemi_294/1
  emi_2084/1 -> cfblk8/Action
  emi_2084/2 -> emi_2082/Action
  emi_2085/1 -> emi_2084/1

== system sampleModel7126_pp_1_1/cfblk253 ==
  cfblk1 : Inport
  cfblk8 : Inport  Port=2
  Action Port : ActionPort  ActionType=then
  cfblk10 : Subsystem  TreatAsAtomicUnit=on
  cfblk{3,11..14,16} (6 alike) : Delay
  cfblk15 : Subsystem  TreatAsAtomicUnit=on
  cfblk4 : Subsystem  TreatAsAtomicUnit=on
  cfblk5 : simulink/Discrete/Transfer Fcn First Order  PoleZ=0.95  ICPrevOutput=0.0  DoSatur=off
      settings: SourceProductName=Simulink
  cfblk6 : DiscreteStateSpace  SampleTime=-1
  cfblk7 : If  SampleTime=1
  cfblk9 : Subsystem  TreatAsAtomicUnit=on
  cyemi_{299..302,312..326} (19 alike) : DataTypeConversion  OutDataTypeStr=double
  emi_1499 : Subsystem  TreatAsAtomicUnit=on
  emi_1501 : If  IfExpression=0 <= u1  SampleTime=[1 0]
  emi_1502 : DataTypeConversion  OutDataTypeStr=double
  emi_713 : Subsystem  TreatAsAtomicUnit=on
  emi_715 : If  IfExpression=0 <= u1  SampleTime=[1 0]
  emi_716 : DataTypeConversion  OutDataTypeStr=double
  cfblk2 : Outport
  wires:
  cfblk6/1 -> cyemi_314/1, cyemi_315/1
  cfblk3/1 -> cyemi_312/1, cyemi_313/1, emi_1502/1
  cfblk5/1 -> cfblk2/1
  cfblk7/1 -> cfblk9/Action
  cfblk7/2 -> cfblk10/Action
  cyemi_299/1 -> cfblk10/1(cfblk1)
  cfblk1/1 -> cyemi_299/1
  cyemi_300/1 -> cfblk10/2(cfblk12)
  cfblk11/1 -> cyemi_300/1, emi_716/1
  cyemi_301/1 -> cfblk10/3(cfblk13)
  cyemi_302/1 -> cfblk10/4(cfblk14)
  cfblk8/1 -> cyemi_302/1
  cyemi_312/1 -> cfblk11/1
  cyemi_313/1 -> cfblk12/1
  cyemi_314/1 -> cfblk13/1
  cyemi_315/1 -> cfblk14/1
  cfblk9/2(cfblk7) -> cyemi_316/1
  cyemi_317/1 -> cfblk16/1
  cyemi_318/1 -> cfblk3/1
  cfblk10/1(cfblk2) -> cyemi_318/1
  cfblk9/4(cfblk9) -> cyemi_319/1
  cyemi_320/1 -> cfblk5/1
  cfblk9/3(cfblk8) -> cyemi_320/1
  cyemi_321/1 -> cfblk6/1
  cfblk9/1(cfblk2) -> cyemi_321/1
  cyemi_322/1 -> cfblk7/1
  cfblk13/1 -> cyemi_322/1
  cyemi_323/1 -> cfblk9/1(cfblk1)
  cfblk16/1 -> cyemi_323/1
  cyemi_324/1 -> cfblk9/2(cfblk4)
  cfblk10/2(cfblk15) -> cyemi_324/1
  cyemi_325/1 -> cfblk9/3(cfblk5)
  cfblk12/1 -> cyemi_325/1
  cyemi_326/1 -> cfblk9/4(cfblk6)
  cfblk14/1 -> cyemi_326/1
  cyemi_316/1 -> cfblk15/1(emi_711)
  cfblk15/1(emi_712) -> cyemi_301/1
  emi_715/1 -> cfblk15/Action
  emi_715/2 -> emi_713/Action
  emi_716/1 -> emi_715/1
  cyemi_319/1 -> cfblk4/1(emi_1497)
  cfblk4/1(emi_1498) -> cyemi_317/1
  emi_1501/1 -> cfblk4/Action
  emi_1501/2 -> emi_1499/Action
  emi_1502/1 -> emi_1501/1

== system sampleModel7126_pp_1_1/cfblk254 ==
  cfblk1 : Inport
  cfblk14 : Inport  Port=2
  cfblk15 : Inport  Port=3
  cfblk16 : Inport  Port=4
  Action Port : ActionPort  ActionType=else
  cfblk10 : simulink/Discrete/Transfer Fcn Lead or Lag  PoleZ=0.95  ZeroZ=0.75  ICPrevOutput=0.0  ICPrevInput=0.0  DoSatur=off
      settings: SourceProductName=Simulink  SourceProductBaseCode=SL
  cfblk11 : DiscreteTransferFcn
  cfblk12 : Delay  ShowEnablePort=on
      settings: InputPortMap=u0,e6
  cfblk13 : simulink/Discrete/Tapped Delay  vinit=0.0  samptime=-1  NumDelays=1  DelayOrder=Oldest  includeCurrent=off
  cfblk3 : DiscreteFilter
  cfblk4 : DiscreteIntegrator  SampleTime=-1  OutDataTypeStr=double  ICPrevOutput=DiscIntNeverNeededParam  ICPrevScaledInput=DiscIntNeverNeededParam
  cfblk5 : simulink/Continuous/PID Controller  Controller=PID  TimeDomain=Discrete-time  SampleTime=-1  IntegratorMethod=Forward Euler  FilterMethod=Forward Euler  Form=Parallel  UseFilter=on  ControllerParametersSource=internal  P=1  I=1  D=0  N=100  InitialConditionSource=internal  InitialConditionForIntegrator=0  InitialConditionForFilter=0  ExternalReset=none  LimitOutput=off  UpperSaturationLimit=inf  LowerSaturationLimit=-inf  LinearizeAsGain=off  AntiWindupMode=none  Kb=1  TrackingMode=off  Kt=1  PParamMin=[]  PParamMax=[]  IParamMin=[]  IParamMax=[]  DParamMin=[]  DParamMax=[]  NParamMin=[]  NParamMax=[]  KbParamMin=[]  KbParamMax=[]  KtParamMin=[]  KtParamMax=[]  POutMin=[]  POutMax=[]  IOutMin=[]  IOutMax=[]  DOutMin=[]  DOutMax=[]  NOutMin=[]  NOutMax=[]  KbOutMin=[]  KbOutMax=[]  KtOutMin=[]  KtOutMax=[]  IntegratorOutMin=[]  IntegratorOutMax=[]  FilterOutMin=[]  FilterOutMax=[]  SumOutMin=[]  SumOutMax=[]  SumI1OutMin=[]  SumI1OutMax=[]  SumI2OutMin=[]  SumI2OutMax=[]  SumI3OutMin=[]  SumI3OutMax=[]  SumDOutMin=[]  SumDOutMax=[]  SaturationOutMin=[]  SaturationOutMax=[]  IntegratorContinuousStateAttributes=''  IntegratorStateMustResolveToSignalObject=off  IntegratorRTWStateStorageClass=Auto  FilterContinuousStateAttributes=''  FilterStateMustResolveToSignalObject=off  FilterRTWStateStorageClass=Auto  DifferentiatorICPrevScaledInput=0  DifferentiatorOutMin=[]  DifferentiatorOutMax=[]  FilterDiffOutCoefMin=[]  FilterDiffOutCoefMax=[]  SumDenOutMin=[]  SumDenOutMax=[]  SumNumOutMin=[]  SumNumOutMax=[]  ReciprocalOutMin=[]  ReciprocalOutMax=[]  DivideOutMin=[]  DivideOutMax=[]  TunerSelectOption=Transfer Function Based (PID Tuner App)
  cfblk6 : Delay  DelayLengthSource=Input port
      settings: InputPortMap=u0,p1
  cfblk7 : simulink/Continuous/PID Controller  Controller=PID  TimeDomain=Discrete-time  SampleTime=-1  IntegratorMethod=Forward Euler  FilterMethod=Forward Euler  Form=Parallel  UseFilter=on  ControllerParametersSource=internal  P=1  I=1  D=0  N=100  InitialConditionSource=internal  InitialConditionForIntegrator=0  InitialConditionForFilter=0  ExternalReset=none  LimitOutput=off  UpperSaturationLimit=inf  LowerSaturationLimit=-inf  LinearizeAsGain=off  AntiWindupMode=none  Kb=1  TrackingMode=off  Kt=1  PParamMin=[]  PParamMax=[]  IParamMin=[]  IParamMax=[]  DParamMin=[]  DParamMax=[]  NParamMin=[]  NParamMax=[]  KbParamMin=[]  KbParamMax=[]  KtParamMin=[]  KtParamMax=[]  POutMin=[]  POutMax=[]  IOutMin=[]  IOutMax=[]  DOutMin=[]  DOutMax=[]  NOutMin=[]  NOutMax=[]  KbOutMin=[]  KbOutMax=[]  KtOutMin=[]  KtOutMax=[]  IntegratorOutMin=[]  IntegratorOutMax=[]  FilterOutMin=[]  FilterOutMax=[]  SumOutMin=[]  SumOutMax=[]  SumI1OutMin=[]  SumI1OutMax=[]  SumI2OutMin=[]  SumI2OutMax=[]  SumI3OutMin=[]  SumI3OutMax=[]  SumDOutMin=[]  SumDOutMax=[]  SaturationOutMin=[]  SaturationOutMax=[]  IntegratorContinuousStateAttributes=''  IntegratorStateMustResolveToSignalObject=off  IntegratorRTWStateStorageClass=Auto  FilterContinuousStateAttributes=''  FilterStateMustResolveToSignalObject=off  FilterRTWStateStorageClass=Auto  DifferentiatorICPrevScaledInput=0  DifferentiatorOutMin=[]  DifferentiatorOutMax=[]  FilterDiffOutCoefMin=[]  FilterDiffOutCoefMax=[]  SumDenOutMin=[]  SumDenOutMax=[]  SumNumOutMin=[]  SumNumOutMax=[]  ReciprocalOutMin=[]  ReciprocalOutMax=[]  DivideOutMin=[]  DivideOutMax=[]  TunerSelectOption=Transfer Function Based (PID Tuner App)
  cfblk8 : DiscreteIntegrator  SampleTime=-1  OutDataTypeStr=double  ICPrevOutput=DiscIntNeverNeededParam  ICPrevScaledInput=DiscIntNeverNeededParam
  cfblk9 : simulink/Discrete/Transfer Fcn Real Zero  ZeroZ=0.75  ICPrevInput=0.0  DoSatur=off
      settings: SourceProductName=Simulink  SourceProductBaseCode=SL
  cyemi_{332..344} (13 alike) : DataTypeConversion  OutDataTypeStr=double
  cfblk2 : Outport
  wires:
  cfblk9/1 -> cfblk2/1
  cyemi_332/1 -> cfblk10/1
  cfblk4/1 -> cyemi_332/1
  cyemi_333/1 -> cfblk11/1
  cfblk7/1 -> cyemi_333/1
  cyemi_334/1 -> cfblk12/1
  cfblk10/1 -> cyemi_334/1
  cyemi_335/1 -> cfblk12/2
  cfblk6/1 -> cyemi_335/1
  cyemi_336/1 -> cfblk13/1
  cfblk14/1 -> cyemi_336/1
  cyemi_337/1 -> cfblk3/1
  cfblk8/1 -> cyemi_337/1
  cyemi_338/1 -> cfblk4/1
  cfblk1/1 -> cyemi_338/1
  cyemi_339/1 -> cfblk5/1
  cfblk13/1 -> cyemi_339/1
  cyemi_340/1 -> cfblk6/1
  cfblk16/1 -> cyemi_340/1
  cyemi_341/1 -> cfblk6/2
  cfblk15/1 -> cyemi_341/1
  cyemi_342/1 -> cfblk7/1
  cfblk3/1 -> cyemi_342/1
  cyemi_343/1 -> cfblk8/1
  cfblk5/1 -> cyemi_343/1
  cyemi_344/1 -> cfblk9/1
  cfblk12/1 -> cyemi_344/1

== system sampleModel7126_pp_1_1/cfblk255 ==
  cfblk1 : Inport
  cfblk9 : Inport  Port=2
  cfblk10 : Inport  Port=3
  cfblk11 : Inport  Port=4
  Action Port : ActionPort  ActionType=then
  cfblk3 : Subsystem  TreatAsAtomicUnit=on
  cfblk4 : DiscreteFir
  cfblk5 : Subsystem  TreatAsAtomicUnit=on
  cfblk6 : Subsystem  TreatAsAtomicUnit=on
  cfblk7 : Delay  ShowEnablePort=on
      settings: InputPortMap=u0,e6
  cfblk8 : simulink/Discrete/Tapped Delay  vinit=0.0  samptime=-1  NumDelays=1  DelayOrder=Oldest  includeCurrent=off
  cyemi_{349..356} (8 alike) : DataTypeConversion  OutDataTypeStr=double
  emi_1794 : Subsystem  TreatAsAtomicUnit=on
  emi_1796 : If  IfExpression=0 <= u1  SampleTime=[1 0]
  emi_1797 : DataTypeConversion  OutDataTypeStr=double
  emi_776 : Subsystem  TreatAsAtomicUnit=on
  emi_778 : If  IfExpression=0 <= u1
  emi_779 : DataTypeConversion  OutDataTypeStr=double
  emi_948 : Subsystem  TreatAsAtomicUnit=on
  emi_950 : If  IfExpression=0 <= u1  SampleTime=[1 0]
  emi_951 : DataTypeConversion  OutDataTypeStr=double
  cfblk2 : Outport
  cfblk12 : Outport  Port=2
  cfblk13 : Outport  Port=3
  wires:
  cfblk7/1 -> cfblk12/1, emi_779/1
  cfblk8/1 -> cyemi_351/1, cyemi_352/1, emi_951/1, emi_1797/1
  cfblk10/1 -> cfblk13/1
  cyemi_350/1 -> cfblk4/1
  cfblk9/1 -> cyemi_353/1
  cyemi_354/1 -> cfblk7/1
  cfblk4/1 -> cyemi_354/1
  cyemi_355/1 -> cfblk7/2
  cfblk1/1 -> cyemi_355/1
  cyemi_356/1 -> cfblk8/1
  cfblk11/1 -> cyemi_356/1
  cyemi_349/1 -> cfblk3/1(emi_774)
  cfblk3/1(emi_775) -> cyemi_350/1
  emi_778/1 -> cfblk3/Action
  emi_778/2 -> emi_776/Action
  emi_779/1 -> emi_778/1
  cyemi_352/1 -> cfblk6/1(emi_945)
  cyemi_353/1 -> cfblk6/2(emi_946)
  cfblk6/1(emi_947) -> cyemi_349/1
  emi_950/1 -> cfblk6/Action
  emi_950/2 -> emi_948/Action
  emi_951/1 -> emi_950/1
  cyemi_351/1 -> cfblk5/1(emi_1792)
  cfblk5/1(emi_1793) -> cfblk2/1
  emi_1796/1 -> cfblk5/Action
  emi_1796/2 -> emi_1794/Action
  emi_1797/1 -> emi_1796/1
